simulink model "PHRControl"  (R2022a)
settings: Solver=FixedStepAuto  StartTime=0.0  StopTime=inf  FixedStep=.005  RelTol=1e-3
model workspace (MAT data in the model file):
  CPR = 10000
  amplitude = 0
  contactTime = 0
  desired_speed = 0
  equilibrium_length = 0
  h = 35
  hip_bend_factor = 0
  hip_fuzz = 0
  initHip = 0.523598775598
  initKnee = -1.0471975512
  k_landing_angle = 0
  k_slip = 0
  knee_bend_factor = 0
  knee_fuzz = 0
  lower_leg_length = 0.15
  max_torque = 8
  r = 1.35
  sample_time = [0 1]
  upper_leg_length = 0.15
  v_des = 0
  z_des = 0
undefined symbols (not defined in the file or in its folder): DiscIntNeverNeededParam, foot_x_flight, foot_y_flight, hasHopped, Hip_Impact_Angle, hip_range, Knee_Impact_Angle, Simscape_Transitions, simTime, SLIP_impact_angle
libraries: slpidlib x16, canmsglib x8, speedgoatlib_IO691 x7, simulink x2, slrealtimeutilitieslib x2
(part 1 of 3)
settings Model: Creator=seanw  LastModifiedBy=seanw
settings SolverCC: ConcurrentTasks=on  PositivePriorityOrder=on
settings OptimizationCC: BlockReduction=off  OptimizeBlockIOStorage=off
settings DebuggingCC: TasksWithSamePriorityMsg=none
settings HardwareCC: ProdBitPerLong=64  ProdLongLongMode=on  ProdHWDeviceType=Intel->x86-64 (Linux 64)
settings RTWCC: Description=Simulink Real-Time  SystemTargetFile=slrealtime.tlc  TemplateMakefile=slrealtime_default_tmf  Toolchain=Simulink Real-Time Toolchain  BuildConfiguration=Specify  CodeExecutionProfiling=on  TargetLang=C++
settings CodeAppCC: MaxIdLength=95

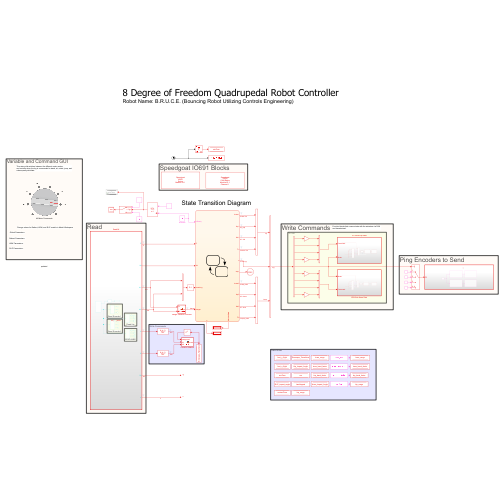
[thumbnail: Simulink's stored preview of the top-level diagram]
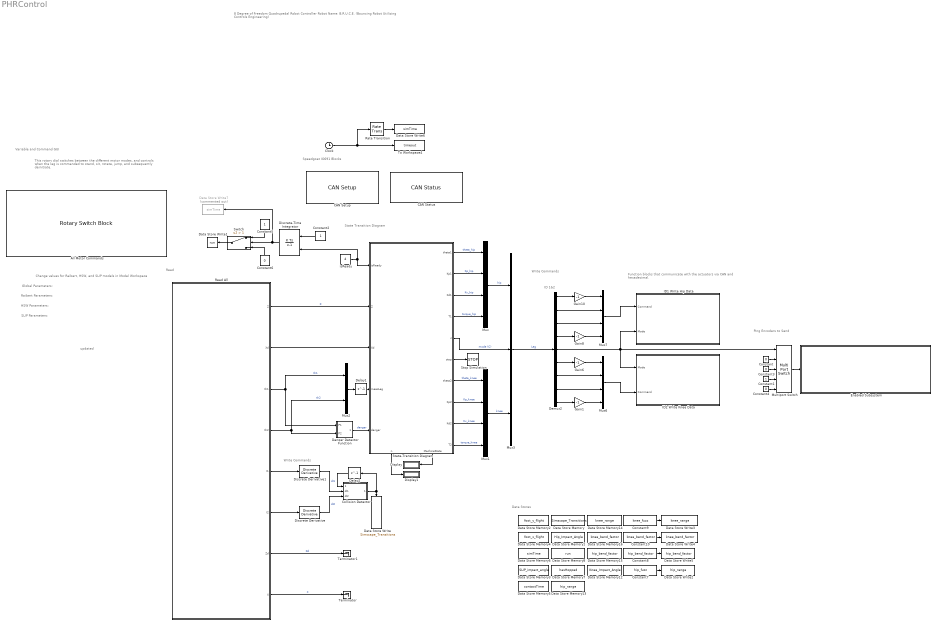
== system PHRControl ==
  note: updated
  note: Write Commands
  note: Data Stores
  note: Global Parameters:
  note: SLIP Parameters:
  note: HSW Parameters:
  note: Raibert Parameters:
  note: Change values for Raibert, HSW, and SLIP models in Model Workspace
  note: Variable and Command GUI
  note: This rotary dial switches between the different motor modes,
      | and controls when the leg is commanded to stand, sit, rotate, jump, and
      | subsequently deinitiate.
  note: Function blocks that communicate with the actuators via CAN
      | and hexadecimal.
  note: Speedgoat IO691 Blocks
  note: State Transition Diagram
  note: ID 1&2
  note: 8 Degree of Freedom Quadrupedal Robot Controller
      | Robot Name: B.R.U.C.E. (Bouncing Robot Utilizing Controls Engineering)
  note: Write Commands
  note: Read
  note: Ping Encoders to Send
  All Motor Commands : RotarySwitchBlock
      settings: Values={{'Zeroing', 'Initiated', 'Stand', 'Raibert', 'HSW', 'SLIP', 'deinit', 'Jump'}, [0 1 2 3 5 6 4 7]}
  "CAN Setup " : speedgoatlib_IO691/Legacy/CAN Setup   moduletype=IO691  id=1  pciSlot=-1  chn1=CAN (HS)  chn2=CAN (HS)  chn3=Disabled  chn4=Disabled  initStruct=[]  termStruct=[]  ArbitrationbdrChn1=1.0 MBaud  ArbitrationManbdrChn1=[2,8,31,8]  FdbdrChn1=5.0 MBaud  FdManbdrChn1=[2,2,5,2]  ArbitrationbdrChn2=1.0 MBaud  ArbitrationManbdrChn2=[2,8,31,8]  FdbdrChn2=5.0 MBaud  FdManbdrChn2=[2,2,5,2]  ArbitrationbdrChn3=1.0 MBaud  ArbitrationManbdrChn3=[2,8,31,8]  FdbdrChn3=5.0 MBaud  FdManbdrChn3=[2,2,5,2]  ArbitrationbdrChn4=1.0 MBaud  ArbitrationManbdrChn4=[2,8,31,8]  FdbdrChn4=5.0 MBaud  FdManbdrChn4=[2,2,5,2]  moduleInitValues=[691 1 -1 -1]
      settings: SourceProductName=Simulink Real-Time: Speedgoat I/O Blockset
  CAN Status : speedgoatlib_IO691/Legacy/CAN Status  moduleId=1  sampleTime=-1  channel=1  busRecovery=Off  arrayOutput=off  controllerCpuLoad=off  controllerLiveCount=off  initModeAct=off  avgBusLoad=off  receiving=off  RxQueueEmpty=off  dataOverrunRcv=off  rxBufferLevel=off  txPending=off  dataOverrunTx=off  txBufferLevel=off  errWarnLimit=off  errPassLimit=off  errBusOff=off  busRecoveryCounter=off  busCouplingErr=off  transceiverErr=off  opMode=off  brp=off  timeSegment1=off  timeSegment2=off  synchronisationJumpWidth=off  dataTSEG1=off  dataTSEG2=off  dataSJW=off  moduleType=691  qtyStatBlk=1  ptIdx=0  isFDMod=0
      settings: SourceProductName=Simulink Real-Time: Speedgoat I/O Blockset
  Clock : Clock
  Collision Detector : MATLAB Function  TreatAsAtomicUnit=on
  Constant{,3..4,6} (4 alike) : Constant  Value=0
  Constant1 : Constant
  Constant10 : Constant  Value=knee_bend_factor
  Constant2 : Constant
  Constant5 : Constant
  Constant7 : Constant  Value=hip_fuzz
  Constant8 : Constant  Value=hip_bend_factor
  Constant9 : Constant  Value=knee_fuzz
  Danger Detector Function : MATLAB Function  TreatAsAtomicUnit=on
  Data Store Memory : DataStoreMemory  DataStoreName=Simscape_Transitions  WriteAfterWriteMsg=warning  ShowAdditionalParam=off  OutDataTypeStr=boolean  Dimensions=1
  Data Store Memory1 : DataStoreMemory  DataStoreName=Hip_Impact_Angle  WriteAfterWriteMsg=warning  ShowAdditionalParam=off  OutDataTypeStr=double
  Data Store Memory12 : DataStoreMemory  DataStoreName=Knee_Impact_Angle  WriteAfterWriteMsg=warning  ShowAdditionalParam=off  OutDataTypeStr=double
  Data Store Memory13 : DataStoreMemory  DataStoreName=hip_range  WriteAfterWriteMsg=warning  ShowAdditionalParam=off  OutDataTypeStr=double
  Data Store Memory14 : DataStoreMemory  DataStoreName=knee_range  WriteAfterWriteMsg=warning  ShowAdditionalParam=off  OutDataTypeStr=double
  Data Store Memory15 : DataStoreMemory  DataStoreName=hip_bend_factor  WriteAfterWriteMsg=warning  ShowAdditionalParam=off  OutDataTypeStr=double
  Data Store Memory16 : DataStoreMemory  DataStoreName=knee_bend_factor  WriteAfterWriteMsg=warning  ShowAdditionalParam=off  OutDataTypeStr=double
  Data Store Memory2 : DataStoreMemory  DataStoreName=foot_y_flight  WriteAfterWriteMsg=warning  ShowAdditionalParam=off  OutDataTypeStr=double
  Data Store Memory3 : DataStoreMemory  DataStoreName=SLIP_impact_angle  WriteAfterWriteMsg=warning  ShowAdditionalParam=off  OutDataTypeStr=double
  Data Store Memory4 : DataStoreMemory  DataStoreName=foot_x_flight  WriteAfterWriteMsg=warning  ShowAdditionalParam=off  OutDataTypeStr=double
  Data Store Memory5 : DataStoreMemory  DataStoreName=contactTime  WriteAfterWriteMsg=warning  ShowAdditionalParam=off  OutDataTypeStr=double
  Data Store Memory6 : DataStoreMemory  DataStoreName=simTime  WriteAfterWriteMsg=warning  ShowAdditionalParam=off  OutDataTypeStr=double
  Data Store Memory7 : DataStoreMemory  DataStoreName=hasHopped  WriteAfterWriteMsg=warning  ShowAdditionalParam=off  OutDataTypeStr=double
  Data Store Memory8 : DataStoreMemory  DataStoreName=run  WriteAfterWriteMsg=warning  ShowAdditionalParam=off  OutDataTypeStr=double
  Data Store Write : DataStoreWrite  DataStoreName=Simscape_Transitions  IndexOptions=Index vector (dialog)  Indices=1  OutputSizes=1
  Data Store Write1 : DataStoreWrite  DataStoreName=run  IndexOptions=Index vector (dialog)  Indices=1  OutputSizes=1
  Data Store Write2 : DataStoreWrite  DataStoreName=hip_range  IndexOptions=Index vector (dialog)  Indices=1  OutputSizes=1
  Data Store Write3 : DataStoreWrite  DataStoreName=knee_range  IndexOptions=Index vector (dialog)  Indices=1  OutputSizes=1
  Data Store Write4 : DataStoreWrite  DataStoreName=knee_bend_factor  IndexOptions=Index vector (dialog)  Indices=1  OutputSizes=1
  Data Store Write5 : DataStoreWrite  DataStoreName=hip_bend_factor  IndexOptions=Index vector (dialog)  Indices=1  OutputSizes=1
  Data Store Write6 : DataStoreWrite  DataStoreName=simTime  IndexOptions=Index vector (dialog)  Indices=1  OutputSizes=1
  Data Store Write7 : DataStoreWrite  Commented=on  DataStoreName=simTime  IndexOptions=Index vector (dialog)  Indices=1  OutputSizes=1
  Delay1 : Delay  DelayLength=1
  Delay2 : Delay  DelayLength=1  InitialCondition=true
  Demux2 : Demux  Outputs=9
  Discrete Derivative : simulink/Discrete/Discrete Derivative  gainval=1.0  ICPrevScaledInput=0.0  OutMin=[]  OutMax=[]  OutDataType=fixdt(1, 16)  OutScaling=2^-10  DoSatur=off
  Discrete Derivative1 : simulink/Discrete/Discrete Derivative  gainval=1.0  ICPrevScaledInput=0.0  OutMin=[]  OutMax=[]  OutDataType=fixdt(1, 16)  OutScaling=2^-10  DoSatur=off
  Discrete-Time Integrator : DiscreteIntegrator  ExternalReset=either  SampleTime=-1  ICPrevOutput=DiscIntNeverNeededParam  ICPrevScaledInput=DiscIntNeverNeededParam
  Display : Display
  Display1 : Display
  Enabled Subsystem : Subsystem  TreatAsAtomicUnit=on
  Gain{1,6,8,10} (4 alike) : Gain  Gain=-1
  ID1 Write Hip Data : Subsystem  TreatAsAtomicUnit=on
  ID2 Write Knee Data : Subsystem  TreatAsAtomicUnit=on
  Multiport Switch : MultiPortSwitch  Inputs=4  DiagnosticForDefault=None  SaturateOnIntegerOverflow=off  InputSameDT=off
  Mux{,1,6..7} (4 alike) : Mux
  Mux2 : Mux  Inputs=2
  Mux3 : Mux  Inputs=3
  Rate Transition : RateTransition
  Read All : Subsystem  TreatAsAtomicUnit=on
  State-Transition Diagram : Stateflow chart  TreatAsAtomicUnit=on
      settings: PortSchema="{\"entries\":[{\"content\":{\"sides\":[{\"content\":{\"connectorIds\":[\"In2\",\"In4\",\"In3\",\"In5\",\"In1\"]},\"type\":\"ConnectorPlacement.EquallySpacedRectSide\",\"uuid\":\"09499f21-f50c-4ce4-914e-8b9942bcc246\"},{\"content\":{\"connectorIds\":[\"Out4\",\"Out9\",\"Out11\",\"Out7\",\"Out6\",\"Out3\",\"Out5\",\"Out10\",\"Out12\",\"Out8\"],\"side\":\"RIGHT\"},\"type\":\"ConnectorPlacement.EquallySpacedRectSide\",\"uuid\":\"b935e908-ace3-4dfb-ad6d-08dfed6ffdb3\"},{\"content\":{\"connectorIds\":[],\"side\":\"TOP\"},\"type\":\"ConnectorPlacement.EquallySpacedRectSide\",\"uuid\":\"4cd7c5d6-1f1f-4a1f-84b4-9b198395645e\"},{\"content\":{\"connectorIds\":[\"Out1\",\"Out2\"],\"side\":\"BOTTOM\"},\"type\":\"ConnectorPlacement.EquallySpacedRectSide\",\"uuid\":\"080199b4-fbf8-4796-9daf-579e3dfa79ae\"}]},\"type\":\"ConnectorPlacement.EquallySpacedConnector\",\"uuid\":\"2dc6a8af-05a8-4f21-87ab-6863f156f450\"}],\"packageUris\":[\"http://schema.mathworks.com/mf0/Connector/R2020b\"],\"version\":\"1.0\"}"
  Stop Simulation : Stop
  Switch : Switch  Criteria=u2 > Threshold  Threshold=1  SaturateOnIntegerOverflow=off  InputSameDT=off
  Terminator : Terminator
  Terminator1 : Terminator
  To Workspace4 : ToWorkspace  VariableName=timeout  SampleTime=-1
  isReady : Constant  Value=4
  wires:
  Clock/1 -> Rate Transition/1, To Workspace4/1
  isReady/1 -> Discrete-Time Integrator/2, State-Transition Diagram/2(isReady)
  State-Transition Diagram/8(T2) -> Mux1/4  "torque_knee"
  State-Transition Diagram/5(theta2) -> Mux1/1  "theta_knee"
  State-Transition Diagram/3(stop) -> Stop Simulation/1
  Mux7/1 -> ID1 Write Hip Data/1(Command)
  Demux2/2 -> Mux7/2
  Demux2/7 -> Mux6/2
  Gain6/1 -> Mux6/1
  State-Transition Diagram/6(c) -> Mux3/2  "mode (C)"
  Gain10/1 -> Mux7/1
  Mux1/1 -> Mux3/3  "knee"
  Mux6/1 -> ID2 Write Knee Data/2(Command)
  Mux3/1 -> Demux2/1  "Leg"
  Danger Detector Function/1(danger) -> State-Transition Diagram/1(danger)  "danger"
  Mux/1 -> Mux3/1  "hip"
  Demux2/1 -> Gain10/1
  Read All/1(Z) -> State-Transition Diagram/4(Z)  "Z"
  Multiport Switch/1 -> Enabled Subsystem/Enable
  Constant/1 -> Multiport Switch/2
  Constant1/1 -> Multiport Switch/4
  Constant3/1 -> Multiport Switch/3
  Constant4/1 -> Multiport Switch/5
  Demux2/3 -> Mux7/3
  Demux2/4 -> Gain8/1
  State-Transition Diagram/10(Kp2) -> Mux1/2  "Kp_knee"
  State-Transition Diagram/12(Kd2) -> Mux1/3  "Kv_knee"
  State-Transition Diagram/4(theta1) -> Mux/1  "theta_hip"
  State-Transition Diagram/9(Kp1) -> Mux/2  "Kp_hip"
  State-Transition Diagram/11(Kd1) -> Mux/3  "Kv_hip"
  State-Transition Diagram/7(T1) -> Mux/4  "torque_hip"
  Gain8/1 -> Mux7/4
  Demux2/5 -> Multiport Switch/1, ID1 Write Hip Data/2(Mode), ID2 Write Knee Data/1(Mode)
  Gain1/1 -> Mux6/4
  Demux2/9 -> Gain1/1
  Demux2/6 -> Gain6/1
  Demux2/8 -> Mux6/3
  Mux2/1 -> Delay1/1
  Delay1/1 -> State-Transition Diagram/5(measLeg)
  State-Transition Diagram/2(MachineState) -> Display/1
  State-Transition Diagram/1(n) -> Display1/1
  Constant2/1 -> Discrete-Time Integrator/1
  Discrete-Time Integrator/1 -> Switch/2, Data Store Write7/1
  Switch/1 -> Data Store Write1/1
  Constant5/1 -> Switch/1
  Constant6/1 -> Switch/3
  Constant7/1 -> Data Store Write2/1
  Constant8/1 -> Data Store Write5/1
  Constant9/1 -> Data Store Write3/1
  Constant10/1 -> Data Store Write4/1
  Collision Detector/1(ground) -> Delay2/1, Data Store Write/1
  Rate Transition/1 -> Data Store Write6/1
  Delay2/1 -> Collision Detector/1(pastground)
  Discrete Derivative1/1 -> Collision Detector/2(dI1)  "dI1"
  Discrete Derivative/1 -> Collision Detector/3(dI2)  "dI2"
  Read All/7(Zd) -> Terminator1/1  "Zd"
  Read All/3(th1) -> Danger Detector Function/1(P1), Mux2/1  "th1"
  Read All/4(th2) -> Mux2/2, Danger Detector Function/2(P2)  "th2"
  Read All/5(I1) -> Discrete Derivative1/1
  Read All/6(I2) -> Discrete Derivative/1
  Read All/8(X) -> Terminator/1  "X"
  Read All/2(Xd) -> State-Transition Diagram/3(Xd)

== system PHRControl/Enabled Subsystem ==
  Enable : EnablePort
  CAN Pack1 : canmsglib/CAN Pack  MsgList=(none)  MsgName=CAN Msg  MsgIDType=Standard (11-bit identifier)  MsgIdentifier=5  MsgLength=0  Remote=off  ApplyMinMax=off  BusOutput=off  SignalInfo={ 'b1', '0', '8', 'LE', 'unsigned', 'Standard', '0', '1', '0', '-Inf', 'Inf'; 'b2', '8', '8', 'LE', 'unsigned', 'Standard', '0', '1', '0', '-Inf', 'Inf'; 'b3', '16', '8', 'LE', 'unsigned', 'Standard', '0', '1', '0', '-Inf', 'Inf'; 'b4', '24', '8', 'LE', 'unsigned', 'Standard', '0', '1', '0', '-Inf', 'Inf'; 'b5', '32', '8', 'LE', 'unsigned', 'Standard', '0', '1', '0', '-Inf', 'Inf'; 'b6', '40', '8', 'LE', 'unsigned', 'Standard', '0', '1', '0', '-Inf', 'Inf'; 'b7', '48', '8', 'LE', 'unsigned', 'Standard', '0', '1', '0', '-Inf', 'Inf'; 'b8', '56', '8', 'LE', 'unsigned', 'Standard', '0', '1', '0', '-Inf', 'Inf' }
      settings: SourceProductBaseCode=XP,ME,VN  DataFormat=raw data
  CAN Pack2 : canmsglib/CAN Pack  MsgList=(none)  MsgName=CAN Msg  MsgIDType=Standard (11-bit identifier)  MsgIdentifier=6  MsgLength=0  Remote=off  ApplyMinMax=off  BusOutput=off  SignalInfo={ 'b1', '0', '8', 'LE', 'unsigned', 'Standard', '0', '1', '0', '-Inf', 'Inf'; 'b2', '8', '8', 'LE', 'unsigned', 'Standard', '0', '1', '0', '-Inf', 'Inf'; 'b3', '16', '8', 'LE', 'unsigned', 'Standard', '0', '1', '0', '-Inf', 'Inf'; 'b4', '24', '8', 'LE', 'unsigned', 'Standard', '0', '1', '0', '-Inf', 'Inf'; 'b5', '32', '8', 'LE', 'unsigned', 'Standard', '0', '1', '0', '-Inf', 'Inf'; 'b6', '40', '8', 'LE', 'unsigned', 'Standard', '0', '1', '0', '-Inf', 'Inf'; 'b7', '48', '8', 'LE', 'unsigned', 'Standard', '0', '1', '0', '-Inf', 'Inf'; 'b8', '56', '8', 'LE', 'unsigned', 'Standard', '0', '1', '0', '-Inf', 'Inf' }
      settings: SourceProductBaseCode=XP,ME,VN  DataFormat=raw data
  CAN Write1 : speedgoatlib_IO691/Legacy/CAN Write  id=1  ts=-1  channel=1  messageType=CAN  BusInput=off  enableStatusPort=off  canType=CAN (HS)  initValues=[691 1 -1 0 1 1 0 0]
      settings: SourceProductName=Simulink Real-Time: Speedgoat I/O Blockset
  CAN Write2 : speedgoatlib_IO691/Legacy/CAN Write  id=1  ts=-1  channel=1  messageType=CAN  BusInput=off  enableStatusPort=off  canType=CAN (HS)  initValues=[691 1 -1 0 1 1 0 0]
      settings: SourceProductName=Simulink Real-Time: Speedgoat I/O Blockset
  Constant : Constant  Value=uint8(1)
  wires:
  Constant/1 -> CAN Pack2/1, CAN Pack1/1
  CAN Pack1/1 -> CAN Write1/1
  CAN Pack2/1 -> CAN Write2/1

== system PHRControl/ID1 Write Hip Data ==
  note: Standard ID Needs to Match Can ID
  note: Converts inputted data to an 8-bit unsigned integer
  Command : Inport
  Mode : Inport  Port=2
  Byte Packing : slrealtimeutilitieslib/Byte Packing  MaskPackedDataType=uint8  MaskUnpackedDataTypes={['uint8']}  MaskAlignment=1
  CAN Pack1 : canmsglib/CAN Pack  MsgList=(none)  MsgName=CAN Msg  MsgIDType=Standard (11-bit identifier)  MsgIdentifier=1  MsgLength=8  Remote=off  ApplyMinMax=off  BusOutput=off  SignalInfo={ 'b1', '0', '8', 'LE', 'unsigned', 'Standard', '0', '1', '0', '-Inf', 'Inf'; 'b2', '8', '8', 'LE', 'unsigned', 'Standard', '0', '1', '0', '-Inf', 'Inf'; 'b3', '16', '8', 'LE', 'unsigned', 'Standard', '0', '1', '0', '-Inf', 'Inf'; 'b4', '24', '8', 'LE', 'unsigned', 'Standard', '0', '1', '0', '-Inf', 'Inf'; 'b5', '32', '8', 'LE', 'unsigned', 'Standard', '0', '1', '0', '-Inf', 'Inf'; 'b6', '40', '8', 'LE', 'unsigned', 'Standard', '0', '1', '0', '-Inf', 'Inf'; 'b7', '48', '8', 'LE', 'unsigned', 'Standard', '0', '1', '0', '-Inf', 'Inf'; 'b8', '56', '8', 'LE', 'unsigned', 'Standard', '0', '1', '0', '-Inf', 'Inf' }
      settings: SourceProductBaseCode=XP,ME,VN  DataFormat=raw data
  CAN Write1 : speedgoatlib_IO691/Legacy/CAN Write  id=1  ts=-1  channel=1  messageType=CAN  BusInput=off  enableStatusPort=off  canType=CAN (HS)  initValues=[691 1 -1 0 1 1 0 0]
      settings: SourceProductName=Simulink Real-Time: Speedgoat I/O Blockset
  Constant : Constant  Value=[0xFF, 0xFF, 0xFF, 0xFF, 0xFF, 0xFF, 0xFF, 0xFE]
  Constant1 : Constant  Value=[0xFF, 0xFF, 0xFF, 0xFF, 0xFF, 0xFF, 0xFF, 0xFC]
  Constant2 : Constant  Value=[0xFF, 0xFF, 0xFF, 0xFF, 0xFF, 0xFF, 0xFF, 0xFD]
  Constant3 : Constant  Value=0
  Demux : Demux
  Multiport Switch : MultiPortSwitch  Inputs=4  DiagnosticForDefault=None  SaturateOnIntegerOverflow=off  InputSameDT=off
  "floats -> bytes" : MATLAB Function  TreatAsAtomicUnit=on
  wires:
  Multiport Switch/1 -> Byte Packing/1
  Demux/1 -> "floats -> bytes"/1(position)  "P_in"
  Constant/1 -> Multiport Switch/2  "Zero"
  Constant2/1 -> Multiport Switch/5  "Deinitiate"
  CAN Pack1/1 -> CAN Write1/1
  Byte Packing/1 -> CAN Pack1/1
  Constant1/1 -> Multiport Switch/3  "Initiate"
  "floats -> bytes"/1(b) -> Multiport Switch/4
  Mode/1 -> Multiport Switch/1  "C1"
  Command/1 -> Demux/1
  Demux/4 -> "floats -> bytes"/5(T_ff)
  Demux/3 -> "floats -> bytes"/4(K_d)
  Demux/2 -> "floats -> bytes"/3(K_p)  "V_in"
  Constant3/1 -> "floats -> bytes"/2(velocity)

== system PHRControl/ID2 Write Knee Data ==
  note: Standard ID Needs to Match Can ID
  Mode : Inport
  Command : Inport  Port=2
  Byte Packing : slrealtimeutilitieslib/Byte Packing  MaskPackedDataType=uint8  MaskUnpackedDataTypes={['uint8']}  MaskAlignment=1
  CAN Pack1 : canmsglib/CAN Pack  MsgList=(none)  MsgName=CAN Msg  MsgIDType=Standard (11-bit identifier)  MsgIdentifier=2  MsgLength=8  Remote=off  ApplyMinMax=off  BusOutput=off  SignalInfo={ 'b1', '0', '8', 'LE', 'unsigned', 'Standard', '0', '1', '0', '-Inf', 'Inf'; 'b2', '8', '8', 'LE', 'unsigned', 'Standard', '0', '1', '0', '-Inf', 'Inf'; 'b3', '16', '8', 'LE', 'unsigned', 'Standard', '0', '1', '0', '-Inf', 'Inf'; 'b4', '24', '8', 'LE', 'unsigned', 'Standard', '0', '1', '0', '-Inf', 'Inf'; 'b5', '32', '8', 'LE', 'unsigned', 'Standard', '0', '1', '0', '-Inf', 'Inf'; 'b6', '40', '8', 'LE', 'unsigned', 'Standard', '0', '1', '0', '-Inf', 'Inf'; 'b7', '48', '8', 'LE', 'unsigned', 'Standard', '0', '1', '0', '-Inf', 'Inf'; 'b8', '56', '8', 'LE', 'unsigned', 'Standard', '0', '1', '0', '-Inf', 'Inf' }
      settings: SourceProductBaseCode=XP,ME,VN  DataFormat=raw data
  CAN Write1 : speedgoatlib_IO691/Legacy/CAN Write  id=1  ts=-1  channel=1  messageType=CAN  BusInput=off  enableStatusPort=off  canType=CAN (HS)  initValues=[691 1 -1 0 1 1 0 0]
      settings: SourceProductName=Simulink Real-Time: Speedgoat I/O Blockset
  Constant : Constant  Value=[0xFF, 0xFF, 0xFF, 0xFF, 0xFF, 0xFF, 0xFF, 0xFE]
  Constant1 : Constant  Value=[0xFF, 0xFF, 0xFF, 0xFF, 0xFF, 0xFF, 0xFF, 0xFC]
  Constant2 : Constant  Value=[0xFF, 0xFF, 0xFF, 0xFF, 0xFF, 0xFF, 0xFF, 0xFD]
  Constant3 : Constant  Value=0
  Demux : Demux
  Multiport Switch : MultiPortSwitch  Inputs=4  DiagnosticForDefault=None  SaturateOnIntegerOverflow=off  InputSameDT=off
  "floats -> bytes" : MATLAB Function  TreatAsAtomicUnit=on
  wires:
  Multiport Switch/1 -> Byte Packing/1
  Demux/1 -> "floats -> bytes"/1(position)  "P_in"
  Constant/1 -> Multiport Switch/2  "Zero"
  Constant2/1 -> Multiport Switch/5  "Deinitiate"
  CAN Pack1/1 -> CAN Write1/1  "CAN msg 2"
  Byte Packing/1 -> CAN Pack1/1
  Constant1/1 -> Multiport Switch/3  "Initiate"
  "floats -> bytes"/1(b) -> Multiport Switch/4
  Mode/1 -> Multiport Switch/1
  Command/1 -> Demux/1
  Demux/4 -> "floats -> bytes"/5(T_ff)
  Demux/3 -> "floats -> bytes"/4(K_d)
  Demux/2 -> "floats -> bytes"/3(K_p)  "V_in"
  Constant3/1 -> "floats -> bytes"/2(velocity)

== system PHRControl/Read All ==
  note: Read Encoder 1
  note: ID 3
  note: ID 4
  note: Read Encoder 2
  note: ID 1
  note: Read Hip
  note: READ KNEE
  note: ID 1&2
  CAN Read : speedgoatlib_IO691/Legacy/CAN Read  id=1  ts=-1  channel=1  messageType=CAN  canType=CAN (HS)  BusOutput=off  initValues=[691 1 -1 0 1 1 0]
      settings: SourceProductName=Simulink Real-Time: Speedgoat I/O Blockset
  Display : Display
  Gain : Gain  Gain=-1
  Gain2 : Gain  Gain=-1
  If Action Subsystem1 : Subsystem  TreatAsAtomicUnit=on
  If Action Subsystem2 : Subsystem  TreatAsAtomicUnit=on
  If Action Subsystem3 : Subsystem  TreatAsAtomicUnit=on
  If Action Subsystem4 : Subsystem  TreatAsAtomicUnit=on
  Terminator{,1..7} (8 alike) : Terminator
  While Iterator : WhileIterator  MaxIters=-1  WhileBlockType=do-while  ResetStates=reset  ShowIterationPort=on
  Z : Outport
  Xd : Outport  Port=2
  th1 : Outport  Port=3
  th2 : Outport  Port=4
  I1 : Outport  Port=5
  I2 : Outport  Port=6
  Zd : Outport  Port=7
  X : Outport  Port=8
  wires:
  CAN Read/1 -> While Iterator/1
  While Iterator/1 -> Display/1
  If Action Subsystem2/1(Z) -> Z/1  "Z"
  If Action Subsystem2/3(Status) -> Terminator7/1
  If Action Subsystem2/2(Zd) -> Zd/1  "Zd"
  If Action Subsystem1/2(Velocity) -> Xd/1  "Xd"
  If Action Subsystem1/3(Status) -> Terminator1/1
  If Action Subsystem1/1(Position) -> X/1  "X"
  If Action Subsystem3/3(Current) -> I1/1  "I_5"
  If Action Subsystem3/2(Velocity) -> Terminator4/1  "V_out"
  If Action Subsystem3/4(ID) -> Terminator6/1  "ID"
  Gain/1 -> th1/1
  If Action Subsystem3/1(Position) -> Gain/1  "P_out"
  If Action Subsystem3/5(Status) -> Terminator2/1
  CAN Read/2 -> If Action Subsystem3/1(In1), If Action Subsystem4/1(In1), If Action Subsystem1/1(In1), If Action Subsystem2/1(In1)
  Gain2/1 -> th2/1
  If Action Subsystem4/5(Status) -> Terminator5/1
  If Action Subsystem4/2(Velocity) -> Terminator/1  "V_out"
  If Action Subsystem4/3(Current) -> I2/1
  If Action Subsystem4/1(Position) -> Gain2/1  "P_out"
  If Action Subsystem4/4(ID) -> Terminator3/1  "ID"

== system PHRControl/State-Transition Diagram/Command1.HSW_Controller ==
  measLeg : Inport
  Xd : Inport  Port=2
  Z : Inport  Port=3
  " Demux " : Demux  Outputs=1
  " Merge " : Merge  Inputs=6
  " Merge 1" : Merge  Inputs=6
  " Merge 2" : Merge  Inputs=6
  " SFunction " : S-Function  Tag=Stateflow S-Function 5  FunctionName=sf_sfun  PortCounts=[3 4]  SFunctionDeploymentMode=off  EnableBusSupport=off
  " Terminator " : Terminator
  Flight : Subsystem
      settings: UndoDeleteFcn=Stateflow.SLINSF.SimulinkMan.restorePreDeleteFcn  PreDeleteFcn=Stateflow.SLINSF.SimulinkMan.removePreDeleteFcn
  HSW : Subsystem
      settings: UndoDeleteFcn=Stateflow.SLINSF.SimulinkMan.restorePreDeleteFcn  PreDeleteFcn=Stateflow.SLINSF.SimulinkMan.removePreDeleteFcn
  Idle : Subsystem
      settings: UndoDeleteFcn=Stateflow.SLINSF.SimulinkMan.restorePreDeleteFcn  PreDeleteFcn=Stateflow.SLINSF.SimulinkMan.removePreDeleteFcn
  Load : Subsystem
      settings: UndoDeleteFcn=Stateflow.SLINSF.SimulinkMan.restorePreDeleteFcn  PreDeleteFcn=Stateflow.SLINSF.SimulinkMan.removePreDeleteFcn
  Unload : Subsystem
      settings: UndoDeleteFcn=Stateflow.SLINSF.SimulinkMan.restorePreDeleteFcn  PreDeleteFcn=Stateflow.SLINSF.SimulinkMan.removePreDeleteFcn
  Machine_State : Outport
  T1 : Outport  Port=2
  T2 : Outport  Port=3
  wires:
  measLeg/1 -> " SFunction "/1, Flight/1(measLeg), Idle/1(measLeg), HSW/1(measLeg)
  Xd/1 -> " SFunction "/2, Flight/2(Xd), HSW/2(Xd)
  Z/1 -> " SFunction "/3, HSW/3(Z)
  " Merge "/1 -> T1/1  "T1"
  " SFunction "/3 -> " Merge "/1  "T1"
  Flight/1(T1) -> " Merge "/2
  " Merge 1"/1 -> T2/1  "T2"
  " SFunction "/4 -> " Merge 1"/1  "T2"
  Flight/2(T2) -> " Merge 1"/2
  " Merge 2"/1 -> Machine_State/1  "Machine_State"
  " SFunction "/2 -> " Merge 2"/1  "Machine_State"
  Flight/3(Machine_State) -> " Merge 2"/2
  Unload/1(T1) -> " Merge "/3
  Unload/2(T2) -> " Merge 1"/3
  Unload/3(Machine_State) -> " Merge 2"/3
  Load/1(T1) -> " Merge "/4
  Load/2(T2) -> " Merge 1"/4
  Load/3(Machine_State) -> " Merge 2"/4
  Idle/1(T1) -> " Merge "/5
  Idle/2(T2) -> " Merge 1"/5
  Idle/3(Machine_State) -> " Merge 2"/5
  HSW/1(T1) -> " Merge "/6
  HSW/2(T2) -> " Merge 1"/6
  HSW/3(Machine_State) -> " Merge 2"/6
  " Demux "/1 -> " Terminator "/1
  " SFunction "/1 -> " Demux "/1

== system PHRControl/State-Transition Diagram/Command1.Raibert ==
  measLeg : Inport
  Xd : Inport  Port=2
  " Demux " : Demux  Outputs=1
  " Merge " : Merge  Inputs=7
  " Merge 1" : Merge  Inputs=7
  " Merge 2" : Merge  Inputs=7
  " SFunction " : S-Function  Tag=Stateflow S-Function 4  FunctionName=sf_sfun  PortCounts=[2 4]  SFunctionDeploymentMode=off  EnableBusSupport=on
  " Terminator " : Terminator
  Compress : Subsystem
      settings: UndoDeleteFcn=Stateflow.SLINSF.SimulinkMan.restorePreDeleteFcn  PreDeleteFcn=Stateflow.SLINSF.SimulinkMan.removePreDeleteFcn
  Flight : Subsystem
      settings: UndoDeleteFcn=Stateflow.SLINSF.SimulinkMan.restorePreDeleteFcn  PreDeleteFcn=Stateflow.SLINSF.SimulinkMan.removePreDeleteFcn
  Idle : Subsystem
      settings: UndoDeleteFcn=Stateflow.SLINSF.SimulinkMan.restorePreDeleteFcn  PreDeleteFcn=Stateflow.SLINSF.SimulinkMan.removePreDeleteFcn
  Load : Subsystem
      settings: UndoDeleteFcn=Stateflow.SLINSF.SimulinkMan.restorePreDeleteFcn  PreDeleteFcn=Stateflow.SLINSF.SimulinkMan.removePreDeleteFcn
  Thrust : Subsystem
      settings: UndoDeleteFcn=Stateflow.SLINSF.SimulinkMan.restorePreDeleteFcn  PreDeleteFcn=Stateflow.SLINSF.SimulinkMan.removePreDeleteFcn
  Unload : Subsystem
      settings: UndoDeleteFcn=Stateflow.SLINSF.SimulinkMan.restorePreDeleteFcn  PreDeleteFcn=Stateflow.SLINSF.SimulinkMan.removePreDeleteFcn
  Machine_State : Outport
  T2 : Outport  Port=2
  T1 : Outport  Port=3
  wires:
  measLeg/1 -> " SFunction "/1, Flight/1(measLeg), Idle/1(measLeg), Compress/1(measLeg)
  Xd/1 -> " SFunction "/2, Flight/2(Xd), Thrust/1(Xd)
  " Merge "/1 -> T1/1  "T1"
  " SFunction "/4 -> " Merge "/1  "T1"
  Flight/1(T1) -> " Merge "/2
  " Merge 1"/1 -> T2/1  "T2"
  " SFunction "/3 -> " Merge 1"/1  "T2"
  Flight/2(T2) -> " Merge 1"/2
  " Merge 2"/1 -> Machine_State/1  "Machine_State"
  " SFunction "/2 -> " Merge 2"/1  "Machine_State"
  Flight/3(Machine_State) -> " Merge 2"/2
  Unload/1(T1) -> " Merge "/3
  Unload/2(T2) -> " Merge 1"/3
  Unload/3(Machine_State) -> " Merge 2"/3
  Load/1(T1) -> " Merge "/4
  Load/2(T2) -> " Merge 1"/4
  Load/3(Machine_State) -> " Merge 2"/4
  Idle/1(T1) -> " Merge "/5
  Idle/2(T2) -> " Merge 1"/5
  Idle/3(Machine_State) -> " Merge 2"/5
  Thrust/1(T1) -> " Merge "/6
  Thrust/2(T2) -> " Merge 1"/6
  Thrust/3(Machine_State) -> " Merge 2"/6
  Compress/1(T1) -> " Merge "/7
  Compress/2(T2) -> " Merge 1"/7
  Compress/3(Machine_State) -> " Merge 2"/7
  " Demux "/1 -> " Terminator "/1
  " SFunction "/1 -> " Demux "/1

== system PHRControl/State-Transition Diagram/Command1.SLIP ==
  measLeg : Inport
  Xd : Inport  Port=2
  " Demux " : Demux  Outputs=1
  " Merge " : Merge  Inputs=6
  " Merge 1" : Merge  Inputs=6
  " Merge 2" : Merge  Inputs=6
  " SFunction " : S-Function  Tag=Stateflow S-Function 3  FunctionName=sf_sfun  PortCounts=[2 5]  SFunctionDeploymentMode=off  EnableBusSupport=on
  " Terminator " : Terminator
  Flight : Subsystem
      settings: UndoDeleteFcn=Stateflow.SLINSF.SimulinkMan.restorePreDeleteFcn  PreDeleteFcn=Stateflow.SLINSF.SimulinkMan.removePreDeleteFcn
  Idle : Subsystem
      settings: UndoDeleteFcn=Stateflow.SLINSF.SimulinkMan.restorePreDeleteFcn  PreDeleteFcn=Stateflow.SLINSF.SimulinkMan.removePreDeleteFcn
  Load : Subsystem
      settings: UndoDeleteFcn=Stateflow.SLINSF.SimulinkMan.restorePreDeleteFcn  PreDeleteFcn=Stateflow.SLINSF.SimulinkMan.removePreDeleteFcn
  Spring : Subsystem
      settings: UndoDeleteFcn=Stateflow.SLINSF.SimulinkMan.restorePreDeleteFcn  PreDeleteFcn=Stateflow.SLINSF.SimulinkMan.removePreDeleteFcn
  Unload : Subsystem
      settings: UndoDeleteFcn=Stateflow.SLINSF.SimulinkMan.restorePreDeleteFcn  PreDeleteFcn=Stateflow.SLINSF.SimulinkMan.removePreDeleteFcn
  Machine_State : Outport
  n : Outport  Port=2
  T1 : Outport  Port=3
  T2 : Outport  Port=4
  wires:
  measLeg/1 -> " SFunction "/1, Flight/1(measLeg), Idle/1(measLeg), Spring/1(measLeg)
  Xd/1 -> " SFunction "/2, Flight/2(Xd)
  " SFunction "/3 -> n/1  "n"
  " Merge "/1 -> T1/1  "T1"
  " SFunction "/4 -> " Merge "/1  "T1"
  Flight/1(T1) -> " Merge "/2
  " Merge 1"/1 -> T2/1  "T2"
  " SFunction "/5 -> " Merge 1"/1  "T2"
  Flight/2(T2) -> " Merge 1"/2
  " Merge 2"/1 -> Machine_State/1  "Machine_State"
  " SFunction "/2 -> " Merge 2"/1  "Machine_State"
  Flight/3(Machine_State) -> " Merge 2"/2
  Unload/1(T1) -> " Merge "/3
  Unload/2(T2) -> " Merge 1"/3
  Unload/3(Machine_State) -> " Merge 2"/3
  Load/1(T1) -> " Merge "/4
  Load/2(T2) -> " Merge 1"/4
  Load/3(Machine_State) -> " Merge 2"/4
  Idle/1(T1) -> " Merge "/5
  Idle/2(T2) -> " Merge 1"/5
  Idle/3(Machine_State) -> " Merge 2"/5
  Spring/1(T1) -> " Merge "/6
  Spring/2(T2) -> " Merge 1"/6
  Spring/3(Machine_State) -> " Merge 2"/6
  " Demux "/1 -> " Terminator "/1
  " SFunction "/1 -> " Demux "/1

== system PHRControl/Read All/If Action Subsystem1 ==
  note: Standard ID Needs to Match Can ID
  In1 : Inport
  CAN Unpack1 : canmsglib/CAN Unpack  MsgList=(none)  MsgName=CAN Msg  MsgIDType=Standard (11-bit identifier)  MsgIdentifier=4  MsgLength=6  SignalInfo={ 'pos', '0', '32', 'LE', 'signed', 'Standard', '0', '1', '0', '-Inf', 'Inf'; 'vel', '32', '16', 'LE', 'signed', 'Standard', '0', '1', '0', '-Inf', 'Inf' }  IDPort=off  TimestampPort=off  ErrorPort=off  RemotePort=off  LengthPort=off  StatusPort=on  ApplyMinMax=off
      settings: SourceProductBaseCode=XP,ME,VN
  Encoder 2 to Vertical Data : MATLAB Function  TreatAsAtomicUnit=on
  Position : Outport
  Velocity : Outport  Port=2
  Status : Outport  Port=3
  wires:
  Encoder 2 to Vertical Data/2(xd) -> Velocity/1
  In1/1 -> CAN Unpack1/1
  Encoder 2 to Vertical Data/1(x) -> Position/1
  CAN Unpack1/3 -> Status/1
  CAN Unpack1/2 -> Encoder 2 to Vertical Data/2(thd2Raw)  "vel"
  CAN Unpack1/1 -> Encoder 2 to Vertical Data/1(th2Raw)  "pos"

== system PHRControl/Read All/If Action Subsystem2 ==
  note: Standard ID Needs to Match Can ID
  In1 : Inport
  CAN Unpack1 : canmsglib/CAN Unpack  MsgList=(none)  MsgName=CAN Msg  MsgIDType=Standard (11-bit identifier)  MsgIdentifier=3  MsgLength=6  SignalInfo={ 'pos', '0', '32', 'LE', 'signed', 'Standard', '0', '1', '0', '-Inf', 'Inf'; 'vel', '32', '16', 'LE', 'signed', 'Standard', '0', '1', '0', '-Inf', 'Inf' }  IDPort=off  TimestampPort=off  ErrorPort=off  RemotePort=off  LengthPort=off  StatusPort=on  ApplyMinMax=off
      settings: SourceProductBaseCode=XP,ME,VN
  Encoder 1 to Vertical Data : MATLAB Function  TreatAsAtomicUnit=on
  Z : Outport
  Zd : Outport  Port=2
  Status : Outport  Port=3
  wires:
  Encoder 1 to Vertical Data/2(zd) -> Zd/1
  In1/1 -> CAN Unpack1/1
  Encoder 1 to Vertical Data/1(z) -> Z/1
  CAN Unpack1/3 -> Status/1
  CAN Unpack1/2 -> Encoder 1 to Vertical Data/2(thd1Raw)  "vel"
  CAN Unpack1/1 -> Encoder 1 to Vertical Data/1(th1Raw)  "pos"

== system PHRControl/Read All/If Action Subsystem3 ==
  note: Standard ID Needs to Match Can ID
  In1 : Inport
  CAN Unpack : canmsglib/CAN Unpack  MsgList=(none)  MsgName=CAN Msg  MsgIDType=Standard (11-bit identifier)  MsgIdentifier=1  MsgLength=6  SignalInfo={ 'position', '16', '16', 'BE', 'unsigned', 'Standard', '0', '1', '0', '0', '65535'; 'velocity', '36', '12', 'BE', 'unsigned', 'Standard', '0', '1', '0', '0', '4095'; 'current', '40', '12', 'BE', 'unsigned', 'Standard', '0', '1', '0', '0', '4095'; 'id', '0', '8', 'BE', 'unsigned', 'Standard', '0', '1', '0', '0', '255' }  IDPort=off  TimestampPort=off  ErrorPort=off  RemotePort=off  LengthPort=off  StatusPort=on  ApplyMinMax=off
      settings: SourceProductBaseCode=XP,ME,VN
  "bytes -> floats" : MATLAB Function  TreatAsAtomicUnit=on
  Position : Outport
  Velocity : Outport  Port=2
  Current : Outport  Port=3
  ID : Outport  Port=4
  Status : Outport  Port=5
  wires:
  CAN Unpack/5 -> Status/1
  CAN Unpack/3 -> "bytes -> floats"/3("I_ff ")
  CAN Unpack/4 -> ID/1
  "bytes -> floats"/2(velocity) -> Velocity/1
  "bytes -> floats"/3(I_ff) -> Current/1
  CAN Unpack/2 -> "bytes -> floats"/2("velocity ")
  In1/1 -> CAN Unpack/1
  CAN Unpack/1 -> "bytes -> floats"/1("position ")
  "bytes -> floats"/1(position) -> Position/1

== system PHRControl/Read All/If Action Subsystem4 ==
  note: Standard ID Needs to Match Can ID
  In1 : Inport
  CAN Unpack : canmsglib/CAN Unpack  MsgList=(none)  MsgName=CAN Msg  MsgIDType=Standard (11-bit identifier)  MsgIdentifier=2  MsgLength=6  SignalInfo={ 'position', '16', '16', 'BE', 'unsigned', 'Standard', '0', '1', '0', '0', '65535'; 'velocity', '36', '12', 'BE', 'unsigned', 'Standard', '0', '1', '0', '0', '4095'; 'current', '40', '12', 'BE', 'unsigned', 'Standard', '0', '1', '0', '0', '4095'; 'id', '0', '8', 'BE', 'unsigned', 'Standard', '0', '1', '0', '0', '255' }  IDPort=off  TimestampPort=off  ErrorPort=off  RemotePort=off  LengthPort=off  StatusPort=on  ApplyMinMax=off
      settings: SourceProductBaseCode=XP,ME,VN
  "bytes -> floats" : MATLAB Function  TreatAsAtomicUnit=on
  Position : Outport
  Velocity : Outport  Port=2
  Current : Outport  Port=3
  ID : Outport  Port=4
  Status : Outport  Port=5
  wires:
  CAN Unpack/5 -> Status/1
  CAN Unpack/1 -> "bytes -> floats"/1("position ")
  CAN Unpack/3 -> "bytes -> floats"/3("I_ff ")
  "bytes -> floats"/1(position) -> Position/1
  CAN Unpack/4 -> ID/1
  "bytes -> floats"/2(velocity) -> Velocity/1
  "bytes -> floats"/3(I_ff) -> Current/1  "I_ff"
  CAN Unpack/2 -> "bytes -> floats"/2("velocity ")
  In1/1 -> CAN Unpack/1

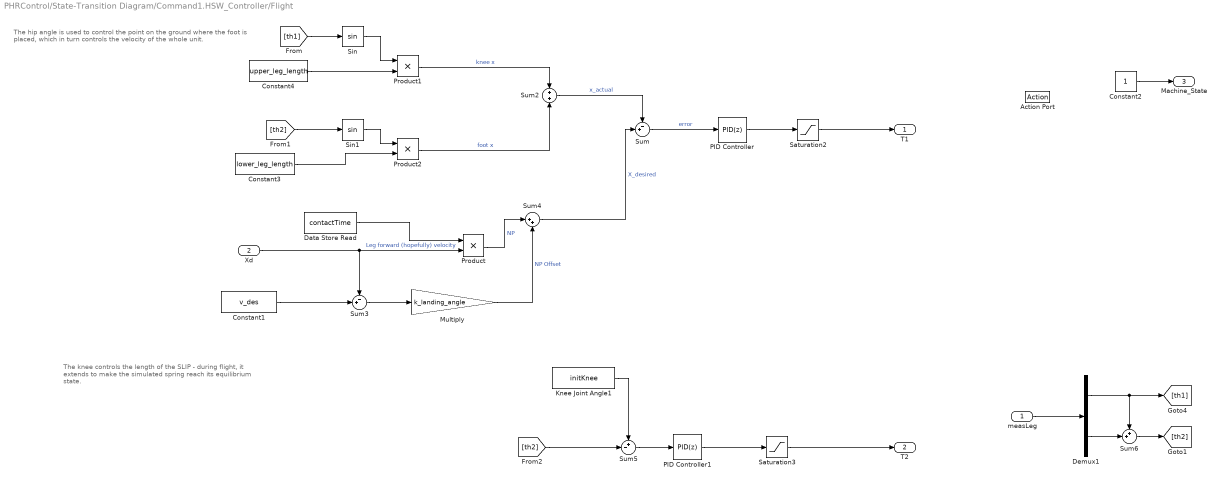
== system PHRControl/State-Transition Diagram/Command1.HSW_Controller/Flight ==
  note: The knee controls the length of the SLIP - during flight, it
      | extends to make the simulated spring reach its equilibrium
      | state.
  note: The hip angle is used to control the point on the ground where the foot is
      | placed, which in turn controls the velocity of the whole unit.
  measLeg : Inport
  Xd : Inport  Port=2
  Action Port : ActionPort
      settings: CopyFcn=Stateflow.SLINSF.SimulinkMan.removeBlockPreDeleteFcn  PreDeleteFcn=Stateflow.SLINSF.SimulinkMan.unsafePredeleteFcn
  Constant1 : Constant  Value=v_des
  Constant2 : Constant
  Constant3 : Constant  Value=lower_leg_length
  Constant4 : Constant  Value=upper_leg_length
  Data Store Read : DataStoreRead  DataStoreName=contactTime  IndexOptions=Index vector (dialog)  Indices=1  OutputSizes=1
  Demux1 : Demux  Outputs=2
  Knee Joint Angle1 : Constant  Value=initKnee
  Multiply : Gain  Gain=k_landing_angle
  PID Controller : slpidlib/PID Controller  Controller=PID  Form=Parallel  TimeDomain=Discrete-time  UseExternalTs=off  SampleTime=-1  IntegratorMethod=Forward Euler  FilterMethod=Forward Euler  ControllerParametersSource=internal  P=50  I=0  UseKiTs=off  D=10  N=100  UseFilter=on  TunerSelectOption=Transfer Function Based (PID Tuner App)  InitialConditionSource=internal  InitialConditionForIntegrator=0  InitialConditionForFilter=0  DifferentiatorICPrevScaledInput=0  ExternalReset=none  TrackingMode=off  Kt=1  LimitOutput=off  SatLimitsSource=internal  UpperSaturationLimit=inf  LowerSaturationLimit=-inf  LinearizeAsGain=on  AntiWindupMode=none  Kb=1  POutMin=[]  POutMax=[]  IOutMin=[]  IOutMax=[]  DOutMin=[]  DOutMax=[]  NOutMin=[]  NOutMax=[]  SumOutMin=[]  SumOutMax=[]  SaturationOutMin=[]  SaturationOutMax=[]  PParamMin=[]  PParamMax=[]  IParamMin=[]  IParamMax=[]  DParamMin=[]  DParamMax=[]  NParamMin=[]  NParamMax=[]  KbParamMin=[]  KbParamMax=[]  KtParamMin=[]  KtParamMax=[]  KbOutMin=[]  KbOutMax=[]  KtOutMin=[]  KtOutMax=[]  IntegratorOutMin=[]  IntegratorOutMax=[]  FilterOutMin=[]  FilterOutMax=[]  SumI1OutMin=[]  SumI1OutMax=[]  SumI2OutMin=[]  SumI2OutMax=[]  SumI3OutMin=[]  SumI3OutMax=[]  SumI4OutMin=[]  SumI4OutMax=[]  SumDOutMin=[]  SumDOutMax=[]  DifferentiatorOutMin=[]  DifferentiatorOutMax=[]  FilterDiffOutCoefMin=[]  FilterDiffOutCoefMax=[]  ReciprocalOutMin=[]  ReciprocalOutMax=[]  SumDenOutMin=[]  SumDenOutMax=[]  SumNumOutMin=[]  SumNumOutMax=[]  DivideOutMin=[]  DivideOutMax=[]  UdiffTsProdOutMin=[]  UdiffTsProdOutMax=[]  NTsProdOutMin=[]  NTsProdOutMax=[]  UintegralTsProdOutMin=[]  UintegralTsProdOutMax=[]  UngainTsProdOutMin=[]  UngainTsProdOutMax=[]  IntegratorContinuousStateAttributes=''  IntegratorStateMustResolveToSignalObject=off  IntegratorRTWStateStorageClass=Auto  FilterContinuousStateAttributes=''  FilterStateMustResolveToSignalObject=off  FilterRTWStateStorageClass=Auto  ParallelPVariant=InternalParameters  IdealPVariant=Disabled  IVariant=InternalParameters  DVariant=InternalParameters  IntegratorVariant=Discrete  SatVariant=Disabled  AWVariant=Passthrough  PCopyVariant=Disabled  TRVariant=Disabled  FdbkBlocksVariant=Forward  IdealPFdbkVariant=Disabled  SatFdbkVariant=Disabled  DerivativeFilterVariant=ForwardEulerFilter  NVariant=InternalParameters  NCopyVariant=Disabled  FilterICVariant=InternalICsFilter  IntegratorICVariant=InternalICs  ExternalResetVariant=Disabled  TRSumVariant=Passthrough  SumFdbkVariant=Disabled  SumVariant=Sum_PID  TsampFilterVariant=InternalTs  TsampNgainVariant=Passthrough  TsampIntegralVariant=Passthrough  ExternalSaturationOutDataTypeStr=Inherit: Same as second input  aMode=0
  PID Controller1 : slpidlib/PID Controller  Controller=PID  Form=Parallel  TimeDomain=Discrete-time  UseExternalTs=off  SampleTime=-1  IntegratorMethod=Forward Euler  FilterMethod=Forward Euler  ControllerParametersSource=internal  P=50  I=0  UseKiTs=off  D=5  N=100  UseFilter=on  TunerSelectOption=Transfer Function Based (PID Tuner App)  InitialConditionSource=internal  InitialConditionForIntegrator=0  InitialConditionForFilter=0  DifferentiatorICPrevScaledInput=0  ExternalReset=none  TrackingMode=off  Kt=1  LimitOutput=off  SatLimitsSource=internal  UpperSaturationLimit=inf  LowerSaturationLimit=-inf  LinearizeAsGain=on  AntiWindupMode=none  Kb=1  POutMin=[]  POutMax=[]  IOutMin=[]  IOutMax=[]  DOutMin=[]  DOutMax=[]  NOutMin=[]  NOutMax=[]  SumOutMin=[]  SumOutMax=[]  SaturationOutMin=[]  SaturationOutMax=[]  PParamMin=[]  PParamMax=[]  IParamMin=[]  IParamMax=[]  DParamMin=[]  DParamMax=[]  NParamMin=[]  NParamMax=[]  KbParamMin=[]  KbParamMax=[]  KtParamMin=[]  KtParamMax=[]  KbOutMin=[]  KbOutMax=[]  KtOutMin=[]  KtOutMax=[]  IntegratorOutMin=[]  IntegratorOutMax=[]  FilterOutMin=[]  FilterOutMax=[]  SumI1OutMin=[]  SumI1OutMax=[]  SumI2OutMin=[]  SumI2OutMax=[]  SumI3OutMin=[]  SumI3OutMax=[]  SumI4OutMin=[]  SumI4OutMax=[]  SumDOutMin=[]  SumDOutMax=[]  DifferentiatorOutMin=[]  DifferentiatorOutMax=[]  FilterDiffOutCoefMin=[]  FilterDiffOutCoefMax=[]  ReciprocalOutMin=[]  ReciprocalOutMax=[]  SumDenOutMin=[]  SumDenOutMax=[]  SumNumOutMin=[]  SumNumOutMax=[]  DivideOutMin=[]  DivideOutMax=[]  UdiffTsProdOutMin=[]  UdiffTsProdOutMax=[]  NTsProdOutMin=[]  NTsProdOutMax=[]  UintegralTsProdOutMin=[]  UintegralTsProdOutMax=[]  UngainTsProdOutMin=[]  UngainTsProdOutMax=[]  IntegratorContinuousStateAttributes=''  IntegratorStateMustResolveToSignalObject=off  IntegratorRTWStateStorageClass=Auto  FilterContinuousStateAttributes=''  FilterStateMustResolveToSignalObject=off  FilterRTWStateStorageClass=Auto  ParallelPVariant=InternalParameters  IdealPVariant=Disabled  IVariant=InternalParameters  DVariant=InternalParameters  IntegratorVariant=Discrete  SatVariant=Disabled  AWVariant=Passthrough  PCopyVariant=Disabled  TRVariant=Disabled  FdbkBlocksVariant=Forward  IdealPFdbkVariant=Disabled  SatFdbkVariant=Disabled  DerivativeFilterVariant=ForwardEulerFilter  NVariant=InternalParameters  NCopyVariant=Disabled  FilterICVariant=InternalICsFilter  IntegratorICVariant=InternalICs  ExternalResetVariant=Disabled  TRSumVariant=Passthrough  SumFdbkVariant=Disabled  SumVariant=Sum_PID  TsampFilterVariant=InternalTs  TsampNgainVariant=Passthrough  TsampIntegralVariant=Passthrough  ExternalSaturationOutDataTypeStr=Inherit: Same as second input  aMode=0
  Product : Product
  Product1 : Product
  Product2 : Product
  Saturation2 : Saturate  UpperLimit=max_torque  LowerLimit=-max_torque
  Saturation3 : Saturate  UpperLimit=max_torque  LowerLimit=-max_torque
  Sin : Trigonometry
  Sin1 : Trigonometry
  Sum : Sum  Inputs=-+|
  Sum2 : Sum  Inputs=+|+
  Sum3 : Sum  Inputs=-+|
  Sum4 : Sum  Inputs=|++
  Sum5 : Sum  Inputs=+-|
  Sum6 : Sum  Inputs=++|
  T1 : Outport
  T2 : Outport  Port=2
  Machine_State : Outport  Port=3
  wires:
  Sum3/1 -> Multiply/1
  Xd/1 -> Product/2, Sum3/1  "Leg forward (hopefully) velocity"
  Sum4/1 -> Sum/2  "X_desired"
  Constant1/1 -> Sum3/2
  PID Controller/1 -> Saturation2/1
  Knee Joint Angle1/1 -> Sum5/1
  PID Controller1/1 -> Saturation3/1
  Saturation2/1 -> T1/1
  Sum5/1 -> PID Controller1/1
  Data Store Read/1 -> Product/1
  Constant2/1 -> Machine_State/1
  Product/1 -> Sum4/1  "NP"
  Sum/1 -> PID Controller/1  "error"
  [th1] -> Sin/1
  Sin/1 -> Product1/1
  Constant4/1 -> Product1/2
  Constant3/1 -> Product2/2
  Sin1/1 -> Product2/1
  Sum2/1 -> Sum/1  "x_actual"
  Product1/1 -> Sum2/1  "knee x"
  Product2/1 -> Sum2/2  "foot x"
  [th2] -> Sin1/1
  Multiply/1 -> Sum4/2  "NP Offset"
  [th2] -> Sum5/2
  Sum6/1 -> [th2]
  Demux1/1 -> Sum6/1, [th1]
  Demux1/2 -> Sum6/2
  measLeg/1 -> Demux1/1
  Saturation3/1 -> T2/1

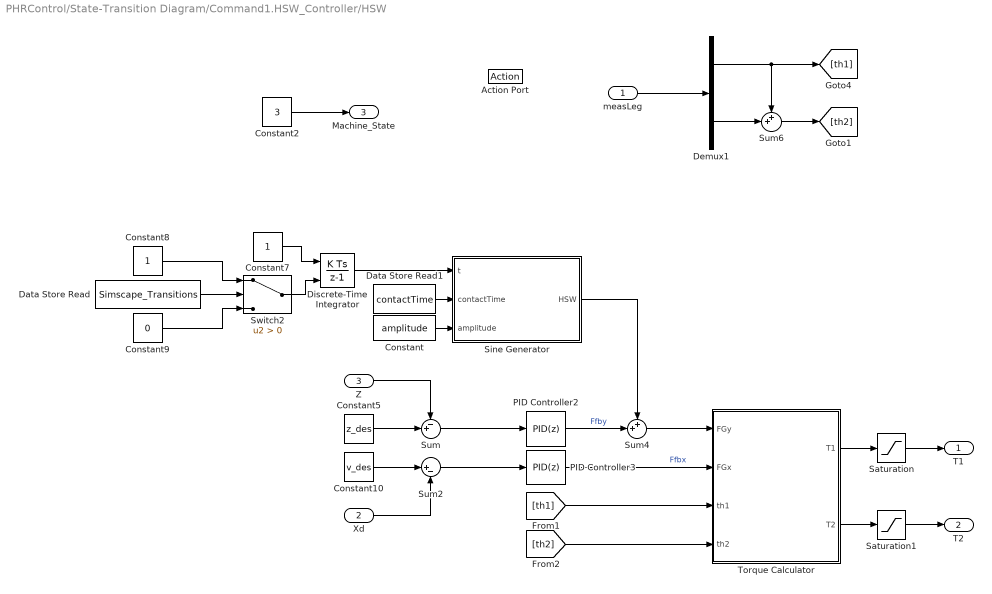
== system PHRControl/State-Transition Diagram/Command1.HSW_Controller/HSW ==
  measLeg : Inport  SampleTime=sample_time
  Xd : Inport  Port=2  SampleTime=sample_time
  Z : Inport  Port=3  SampleTime=sample_time
  Action Port : ActionPort
      settings: CopyFcn=Stateflow.SLINSF.SimulinkMan.removeBlockPreDeleteFcn  PreDeleteFcn=Stateflow.SLINSF.SimulinkMan.unsafePredeleteFcn
  Constant : Constant  Value=amplitude
  Constant10 : Constant  Value=v_des
  Constant2 : Constant  Value=3
  Constant5 : Constant  Value=z_des
  Constant7 : Constant
  Constant8 : Constant
  Constant9 : Constant  Value=0
  Data Store Read : DataStoreRead  DataStoreName=Simscape_Transitions  IndexOptions=Index vector (dialog)  Indices=1  OutputSizes=1
  Data Store Read1 : DataStoreRead  DataStoreName=contactTime  IndexOptions=Index vector (dialog)  Indices=1  OutputSizes=1
  Demux1 : Demux  Outputs=2
  Discrete-Time Integrator : DiscreteIntegrator  ExternalReset=rising  SampleTime=-1  ICPrevOutput=DiscIntNeverNeededParam  ICPrevScaledInput=DiscIntNeverNeededParam
  PID Controller2 : slpidlib/PID Controller  Controller=PID  Form=Parallel  TimeDomain=Discrete-time  UseExternalTs=off  SampleTime=-1  IntegratorMethod=Forward Euler  FilterMethod=Forward Euler  ControllerParametersSource=internal  P=50  I=0  UseKiTs=off  D=0  N=100  UseFilter=on  TunerSelectOption=Transfer Function Based (PID Tuner App)  InitialConditionSource=internal  InitialConditionForIntegrator=0  InitialConditionForFilter=0  DifferentiatorICPrevScaledInput=0  ExternalReset=none  TrackingMode=off  Kt=1  LimitOutput=off  SatLimitsSource=internal  UpperSaturationLimit=inf  LowerSaturationLimit=-inf  LinearizeAsGain=on  AntiWindupMode=none  Kb=1  POutMin=[]  POutMax=[]  IOutMin=[]  IOutMax=[]  DOutMin=[]  DOutMax=[]  NOutMin=[]  NOutMax=[]  SumOutMin=[]  SumOutMax=[]  SaturationOutMin=[]  SaturationOutMax=[]  PParamMin=[]  PParamMax=[]  IParamMin=[]  IParamMax=[]  DParamMin=[]  DParamMax=[]  NParamMin=[]  NParamMax=[]  KbParamMin=[]  KbParamMax=[]  KtParamMin=[]  KtParamMax=[]  KbOutMin=[]  KbOutMax=[]  KtOutMin=[]  KtOutMax=[]  IntegratorOutMin=[]  IntegratorOutMax=[]  FilterOutMin=[]  FilterOutMax=[]  SumI1OutMin=[]  SumI1OutMax=[]  SumI2OutMin=[]  SumI2OutMax=[]  SumI3OutMin=[]  SumI3OutMax=[]  SumI4OutMin=[]  SumI4OutMax=[]  SumDOutMin=[]  SumDOutMax=[]  DifferentiatorOutMin=[]  DifferentiatorOutMax=[]  FilterDiffOutCoefMin=[]  FilterDiffOutCoefMax=[]  ReciprocalOutMin=[]  ReciprocalOutMax=[]  SumDenOutMin=[]  SumDenOutMax=[]  SumNumOutMin=[]  SumNumOutMax=[]  DivideOutMin=[]  DivideOutMax=[]  UdiffTsProdOutMin=[]  UdiffTsProdOutMax=[]  NTsProdOutMin=[]  NTsProdOutMax=[]  UintegralTsProdOutMin=[]  UintegralTsProdOutMax=[]  UngainTsProdOutMin=[]  UngainTsProdOutMax=[]  IntegratorContinuousStateAttributes=''  IntegratorStateMustResolveToSignalObject=off  IntegratorRTWStateStorageClass=Auto  FilterContinuousStateAttributes=''  FilterStateMustResolveToSignalObject=off  FilterRTWStateStorageClass=Auto  ParallelPVariant=InternalParameters  IdealPVariant=Disabled  IVariant=InternalParameters  DVariant=InternalParameters  IntegratorVariant=Discrete  SatVariant=Disabled  AWVariant=Passthrough  PCopyVariant=Disabled  TRVariant=Disabled  FdbkBlocksVariant=Forward  IdealPFdbkVariant=Disabled  SatFdbkVariant=Disabled  DerivativeFilterVariant=ForwardEulerFilter  NVariant=InternalParameters  NCopyVariant=Disabled  FilterICVariant=InternalICsFilter  IntegratorICVariant=InternalICs  ExternalResetVariant=Disabled  TRSumVariant=Passthrough  SumFdbkVariant=Disabled  SumVariant=Sum_PID  TsampFilterVariant=InternalTs  TsampNgainVariant=Passthrough  TsampIntegralVariant=Passthrough  ExternalSaturationOutDataTypeStr=Inherit: Same as second input  aMode=0
  PID Controller3 : slpidlib/PID Controller  Controller=PID  Form=Parallel  TimeDomain=Discrete-time  UseExternalTs=off  SampleTime=-1  IntegratorMethod=Forward Euler  FilterMethod=Forward Euler  ControllerParametersSource=internal  P=50  I=0  UseKiTs=off  D=0  N=100  UseFilter=on  TunerSelectOption=Transfer Function Based (PID Tuner App)  InitialConditionSource=internal  InitialConditionForIntegrator=0  InitialConditionForFilter=0  DifferentiatorICPrevScaledInput=0  ExternalReset=none  TrackingMode=off  Kt=1  LimitOutput=off  SatLimitsSource=internal  UpperSaturationLimit=inf  LowerSaturationLimit=-inf  LinearizeAsGain=on  AntiWindupMode=none  Kb=1  POutMin=[]  POutMax=[]  IOutMin=[]  IOutMax=[]  DOutMin=[]  DOutMax=[]  NOutMin=[]  NOutMax=[]  SumOutMin=[]  SumOutMax=[]  SaturationOutMin=[]  SaturationOutMax=[]  PParamMin=[]  PParamMax=[]  IParamMin=[]  IParamMax=[]  DParamMin=[]  DParamMax=[]  NParamMin=[]  NParamMax=[]  KbParamMin=[]  KbParamMax=[]  KtParamMin=[]  KtParamMax=[]  KbOutMin=[]  KbOutMax=[]  KtOutMin=[]  KtOutMax=[]  IntegratorOutMin=[]  IntegratorOutMax=[]  FilterOutMin=[]  FilterOutMax=[]  SumI1OutMin=[]  SumI1OutMax=[]  SumI2OutMin=[]  SumI2OutMax=[]  SumI3OutMin=[]  SumI3OutMax=[]  SumI4OutMin=[]  SumI4OutMax=[]  SumDOutMin=[]  SumDOutMax=[]  DifferentiatorOutMin=[]  DifferentiatorOutMax=[]  FilterDiffOutCoefMin=[]  FilterDiffOutCoefMax=[]  ReciprocalOutMin=[]  ReciprocalOutMax=[]  SumDenOutMin=[]  SumDenOutMax=[]  SumNumOutMin=[]  SumNumOutMax=[]  DivideOutMin=[]  DivideOutMax=[]  UdiffTsProdOutMin=[]  UdiffTsProdOutMax=[]  NTsProdOutMin=[]  NTsProdOutMax=[]  UintegralTsProdOutMin=[]  UintegralTsProdOutMax=[]  UngainTsProdOutMin=[]  UngainTsProdOutMax=[]  IntegratorContinuousStateAttributes=''  IntegratorStateMustResolveToSignalObject=off  IntegratorRTWStateStorageClass=Auto  FilterContinuousStateAttributes=''  FilterStateMustResolveToSignalObject=off  FilterRTWStateStorageClass=Auto  ParallelPVariant=InternalParameters  IdealPVariant=Disabled  IVariant=InternalParameters  DVariant=InternalParameters  IntegratorVariant=Discrete  SatVariant=Disabled  AWVariant=Passthrough  PCopyVariant=Disabled  TRVariant=Disabled  FdbkBlocksVariant=Forward  IdealPFdbkVariant=Disabled  SatFdbkVariant=Disabled  DerivativeFilterVariant=ForwardEulerFilter  NVariant=InternalParameters  NCopyVariant=Disabled  FilterICVariant=InternalICsFilter  IntegratorICVariant=InternalICs  ExternalResetVariant=Disabled  TRSumVariant=Passthrough  SumFdbkVariant=Disabled  SumVariant=Sum_PID  TsampFilterVariant=InternalTs  TsampNgainVariant=Passthrough  TsampIntegralVariant=Passthrough  ExternalSaturationOutDataTypeStr=Inherit: Same as second input  aMode=0
  Saturation : Saturate  UpperLimit=max_torque  LowerLimit=-max_torque
  Saturation1 : Saturate  UpperLimit=max_torque  LowerLimit=-max_torque
  Sine Generator : MATLAB Function  TreatAsAtomicUnit=on
  Sum : Sum  Inputs=-+|
  Sum2 : Sum  Inputs=|+-
  Sum4 : Sum  Inputs=++|
  Sum6 : Sum  Inputs=++|
  Switch2 : Switch  Criteria=u2 > Threshold  SaturateOnIntegerOverflow=off  InputSameDT=off
  Torque Calculator : MATLAB Function  TreatAsAtomicUnit=on
  T1 : Outport  SampleTime=sample_time
  T2 : Outport  Port=2  SampleTime=sample_time
  Machine_State : Outport  Port=3  SampleTime=sample_time
  wires:
  Constant2/1 -> Machine_State/1
  PID Controller3/1 -> Torque Calculator/2(FGx)  "Ffbx"
  Sum/1 -> PID Controller2/1
  Constant10/1 -> Sum2/1
  Switch2/1 -> Discrete-Time Integrator/2
  Sum2/1 -> PID Controller3/1
  Torque Calculator/1(T1) -> Saturation/1
  [th1] -> Torque Calculator/3(th1)
  Constant5/1 -> Sum/2
  Data Store Read/1 -> Switch2/2
  Discrete-Time Integrator/1 -> Sine Generator/1(t)
  Constant9/1 -> Switch2/3
  Constant8/1 -> Switch2/1
  [th2] -> Torque Calculator/4(th2)
  Sum4/1 -> Torque Calculator/1(FGy)
  Constant7/1 -> Discrete-Time Integrator/1
  PID Controller2/1 -> Sum4/2  "Ffby"
  Sine Generator/1(HSW) -> Sum4/1
  Data Store Read1/1 -> Sine Generator/2(contactTime)
  Constant/1 -> Sine Generator/3(amplitude)
  Sum6/1 -> [th2]
  Demux1/2 -> Sum6/2
  Demux1/1 -> Sum6/1, [th1]
  measLeg/1 -> Demux1/1
  Xd/1 -> Sum2/2
  Saturation/1 -> T1/1
  Torque Calculator/2(T2) -> Saturation1/1
  Saturation1/1 -> T2/1
  Z/1 -> Sum/1
